simulink model "ATOM_simple_planning_simulator"  (R2026a)
settings: Solver=ode4  StopTime=50  FixedStep=0.01
StopFcn:
  | if exist('costmap_active','var') && ...
  |    exist('vehicle','var') && ...
  |    exist('parking_path','var') && ...
  |    ~isempty(parking_path)
  | 
  |     plotPlan(costmap_active, vehicle, parking_path);
  | else
  |     warning('No valid parking path is available for plotting.');
  | end
model workspace (MAT data in the model file):
  vehicle : object (value not decoded)
symbols that are objects in the model workspace (value not decoded): vehicle
undefined symbols (not defined in the file or in its folder): delta_f_LUT, gain4WS_LUT, k_ref_LUT, kappa_gain_BP, Ki, Kp, lateral, longitudinal, planning_validator, rr_gain_BP, rr_LUT, stanley, velocity_smoother
libraries: slpidlib x1, simulink x1
(part 7 of 7)

== matlab function ATOM_simple_planning_simulator/Plot vehicle1/SetStanleyTrajectory/Resample Trajectory ==
  data: trajectory_in input Bus: TrajectoryDataBus; trajectory_out output Bus: TrajectoryDataBus; resample_interval_dist input; nearest_seg_idx input; ego_offset_to_segment input
function trajectory_out = resampleTrajectoryByDistance( ...
    trajectory_in, ...
    resample_interval_dist, ...
    nearest_seg_idx, ...
    ego_offset_to_segment)


%% ============================================================
% RESAMPLE TRAJECTORY BY ARC LENGTH
%
% Equivalent to:
%
% MPCUtils::resampleMPCTrajectoryByDistance()
%
% Adapted for Stanley controller.
%
% Unlike MPC:
% - no MPCTrajectory conversion
% - no curvature resampling
% - no optimization variables
%
% The trajectory is directly interpolated in arc length.
%
% ATTENTION:
% 
% Resampling is not actuated in Simulink since in/out buses present fixed sizes.
% See NOTE at the end of this function.
%
% =============================================================


% N = length(trajectory_in.pose.position.x);
% 
% 
% if N < 2
% 
%     trajectory_out = trajectory_in;
%     return
% 
% end
% 
% 
% 
% %% ============================================================
% % Compute arc length
% % =============================================================
% 
% x = trajectory_in.pose.position.x;
% y = trajectory_in.pose.position.y;
% 
% 
% arc_length = zeros(N,1);
% 
% 
% for i = 2:N
% 
%     dx = x(i)-x(i-1);
%     dy = y(i)-y(i-1);
% 
%     arc_length(i)= ...
%         arc_length(i-1)+sqrt(dx^2+dy^2);
% 
% end
% 
% 
% 
% if isempty(arc_length)
% 
%     trajectory_out = trajectory_in;
%     return
% 
% end
% 
% 
% 
% %% ============================================================
% % Ego position along trajectory
% %
% % Equivalent to:
% %
% % input_arclength(nearest_seg_idx)
% % + ego_offset_to_segment
% %
% % =============================================================
% 
% 
% ego_s = arc_length(nearest_seg_idx) ...
%         + ego_offset_to_segment;
% 
% 
% ego_s = min(max(ego_s,0),arc_length(end));
% 
% 
% 
% %% ============================================================
% % Generate resampling points
% %
% % Same strategy as Autoware:
% % - backward from ego
% % - forward from ego
% %
% % =============================================================
% 
% 
% output_s = [];
% 
% 
% % backward direction
% 
% s = ego_s;
% 
% while s >= 0
% 
%     output_s = [s output_s]; %#ok<AGROW>
% 
%     s = s - resample_interval_dist;
% 
% end
% 
% 
% 
% % forward direction
% 
% s = ego_s + resample_interval_dist;
% 
% 
% while s < arc_length(end)
% 
%     output_s(end+1)=s; % #ok<AGROW>
% 
%     s = s + resample_interval_dist;
% 
% end
% 
% 
% 
% %% ============================================================
% % Interpolation
% % =============================================================
% 
% 
% x_new = interp1( ...
%     arc_length,...
%     x,...
%     output_s,...
%     'linear');
% 
% 
% 
% y_new = interp1( ...
%     arc_length,...
%     y,...
%     output_s,...
%     'linear');
% 
% 
% 
% z = trajectory_in.pose.position.z;
% 
% z_new = interp1( ...
%     arc_length,...
%     z,...
%     output_s,...
%     'linear');
% 
% 
% 
% %% ============================================================
% % Quaternion / yaw interpolation
% %
% % Stanley works with yaw.
% % Therefore interpolate yaw and rebuild quaternion.
% %
% % =============================================================
% 
% 
% yaw = QuaternionToYaw( ...
%     trajectory_in.pose.orientation.qx,...
%     trajectory_in.pose.orientation.qy,...
%     trajectory_in.pose.orientation.qz,...
%     trajectory_in.pose.orientation.qw);
% 
% 
% 
% % avoid discontinuity
% 
% yaw = unwrap(yaw);
% 
% 
% 
% yaw_new = interp1( ...
%     arc_length,...
%     yaw,...
%     output_s,...
%     'linear');
% 
% 
% 
% %% ============================================================
% % Velocity interpolation
% %
% % Autoware uses linear interpolation
% % =============================================================
% 
% 
% vel_new = interp1( ...
%     arc_length,...
%     trajectory_in.longitudinal_velocity_mps,...
%     output_s,...
%     'linear');
% 
% 
% 
% lat_vel_new = interp1( ...
%     arc_length,...
%     trajectory_in.lateral_velocity_mps,...
%     output_s,...
%     'linear');
% 
% 
% 
% acc_new = interp1( ...
%     arc_length,...
%     trajectory_in.acceleration_mps2,...
%     output_s,...
%     'linear');
% 
% 
% 
% %% ============================================================
% % Build output structure
% % =============================================================
% 
% 
% M = length(output_s);
% 
% 
% trajectory_out.pose.position.x = x_new;
% trajectory_out.pose.position.y = y_new;
% trajectory_out.pose.position.z = z_new;
% 
% 
% 
% [qx,qy,qz,qw] = yawToQuaternion(yaw_new);
% 
% 
% 
% trajectory_out.pose.orientation.qx = qx;
% trajectory_out.pose.orientation.qy = qy;
% trajectory_out.pose.orientation.qz = qz;
% trajectory_out.pose.orientation.qw = qw;
% 
% 
% 
% trajectory_out.longitudinal_velocity_mps = vel_new;
% 
% trajectory_out.lateral_velocity_mps = lat_vel_new;
% 
% trajectory_out.acceleration_mps2 = acc_new;
% 
% 
% 
% % steering values are kept
% 
% trajectory_out.front_wheel_angle_rad = ...
%     interp1( ...
%     arc_length,...
%     trajectory_in.front_wheel_angle_rad,...
%     output_s,...
%     'linear');
% 
% 
% trajectory_out.rear_wheel_angle_rad = ...
%     interp1( ...
%     arc_length,...
%     trajectory_in.rear_wheel_angle_rad,...
%     output_s,...
%     'linear');
% 
% 


%% ============================================================
% NOTE (Simulink Implementation)
%
% The trajectory resampling algorithm reported above is equivalent
% to the implementation adopted by Autoware.
%
% However, the main objective of the present work is the development
% and validation of the 4WS Stanley Controller rather than the
% trajectory preprocessing module.
%
% Since Simulink requires fixed-size bus signals, the resampled
% trajectory is not generated in the simulation model.
%
% The original input trajectory is therefore directly propagated to
% the controller, preserving its fixed dimension and avoiding the
% introduction of variable-length signals.
%
% Consequently, the following assignment overwrites the resampled
% trajectory computed above.
%
% ============================================================

trajectory_out = trajectory_in;

end

== matlab function ATOM_simple_planning_simulator/Plot vehicle1/SetStanleyTrajectory/calcLongOffsetToSegment ==
  data: seg_idx input; ego_pose input; trajectory input Bus: TrajectoryDataBus; ego_offset_to_segment output
function ego_offset_to_segment = calcLongOffsetToSegment(seg_idx, ego_pose, trajectory)

ego_offset_to_segment = calcLongitudinalOffsetToSegment(trajectory, seg_idx, ego_pose);

end

== matlab function ATOM_simple_planning_simulator/Plot vehicle1/SetStanleyTrajectory/findFirstNearestSegmentIndexWithSoftConstraints ==
  data: trajectory input; dist_threshold input; yaw_threshold input; nearest_seg_idx output; pose input
function nearest_seg_idx = findNearestSegmentIndexWithSoftConstraints( ...
    trajectory, dist_threshold, yaw_threshold, pose)


%% Step 1:
% Find nearest point index

nearest_idx = findFirstNearestIndexWithSoftConstraints( ...
    trajectory, ...
    pose, ...
    dist_threshold, ...
    yaw_threshold);


N = length(trajectory.pose.position.x);


%% Step 2:
% Convert point index into segment index

% First point
if nearest_idx == 1

    nearest_seg_idx = 1;
    return

end


% Last point
if nearest_idx == N

    nearest_seg_idx = N-1;
    return

end



%% Step 3:
% Determine whether ego lies before or after nearest point
%
% Equivalent to Autoware:
%
% signed_length =
% calcLongitudinalOffsetToSegment(points,
%                                 nearest_idx,
%                                 pose.position)


signed_length = calcLongitudinalOffsetToSegment( ...
    trajectory,...
    nearest_idx,...
    pose);



%% Step 4:
% Choose segment

if signed_length <= 0

    % ego is before nearest point
    %
    % Autoware:
    % return nearest_idx - 1;

    nearest_seg_idx = nearest_idx - 1;


else

    % ego is after nearest point
    %
    % Autoware:
    % return nearest_idx;

    nearest_seg_idx = nearest_idx;

end


end

== matlab function ATOM_simple_planning_simulator/Parking Scenario/MATLAB Function ==
  data: segment_done input; segment_request output; segment_count input; maneuver_complete output
function [segment_request, maneuver_complete] = ...
    segmentManager(segment_done, segment_count)
%SEGMENTMANAGER
% Advance exactly once when the current segment is completed.

persistent active_segment previous_done complete_latched

if isempty(active_segment)
    active_segment  = 1.0;
    previous_done   = false;
    complete_latched = false;
end

% Convert the inputs into known scalar types.
done_now = logical(segment_done);
count = max(0.0, floor(double(segment_count)));

% Protect against an active index larger than the available count.
if count > 0 && active_segment > count
    active_segment = count;
end

% Detect only the transition from not-done to done.
done_rising_edge = done_now && ~previous_done;

if done_rising_edge && count > 0

    if active_segment < count

        % Another segment exists.
        active_segment = active_segment + 1.0;

    else

        % The final segment has been completed.
        complete_latched = true;

    end
end

previous_done = done_now;

segment_request  = active_segment;
maneuver_complete = complete_latched;
end

== matlab function ATOM_simple_planning_simulator/parking_velocity_smoother/MATLAB Function ==
  data: trajectory_in input Bus: TrajectoryDataBus size=1; trajectory_out output Bus: TrajectoryDataBus size=1
function trajectory_out = parkingVelocitySmoother(trajectory_in)
%#codegen
%
% Generate the longitudinal velocity and acceleration reference
% for one forward or reverse parking segment.

% Preserve all fields of the original trajectory bus.
trajectory_out = trajectory_in;

% The parking trajectory contains exactly 100 points.
N = 100;

%% 1. Velocity-profile parameters

v_max       = 2.00;   % desired maximum parking speed [m/s]
a_accel_max = 1.00;   % from velocity_smoother.max_acc
% Plan the trajectory using gentler braking than the controller can
% physically command. The remaining 0.50 m/s^2 provides correction margin
% for tracking error, actuator delay, and acceleration lag.
a_decel_max = 0.50;   % planned braking magnitude [m/s^2]

% Existing lateral-acceleration limit from velocity_smoother_params.m.
a_lat_max = 1.00;     % maximum lateral acceleration [m/s^2]

% Existing curvature-calculation distance from
% velocity_smoother_params.m.
curvature_calculation_distance = 2.00;   % [m]

%% 2. Read the trajectory data

px = trajectory_in.pose.position.x;
py = trajectory_in.pose.position.y;

rear_angle = trajectory_in.rear_wheel_angle_rad;

% At this stage, the incoming velocity is used only to determine
% whether the segment is forward or reverse.
raw_velocity = trajectory_in.longitudinal_velocity_mps;

%% 3. Determine the segment direction

% Default to forward if no nonzero direction can be found.
gear = 1.0;

for k = 1:N
    if abs(raw_velocity(k)) > 1e-6
        gear = sign(raw_velocity(k));
        break;
    end
end

%% 4. Calculate distance between consecutive trajectory points

ds = zeros(N-1,1);
path_length = 0.0;

for k = 1:N-1
    dx = px(k+1) - px(k);
    dy = py(k+1) - py(k);

    ds(k) = hypot(dx,dy);
    path_length = path_length + ds(k);
end

%% 5. Calculate trajectory curvature

% pathToTrajectory resamples the segment at approximately equal
% distances, so an index separation can represent the requested
% curvature-calculation distance.

point_interval = path_length / (N-1);

idx_dist = 1;

if point_interval > 1e-6
    idx_dist = floor( ...
        curvature_calculation_distance / point_interval);
end

% Three curvature points must remain inside the trajectory.
max_idx_dist = floor((N-1)/2);

idx_dist = max(1,min(idx_dist,max_idx_dist));

curvature = zeros(N,1);

for k = 2:N-1

    idx_prev = k - min(idx_dist,k-1);
    idx_next = k + min(idx_dist,N-k);

    x1 = px(idx_prev);
    y1 = py(idx_prev);

    x2 = px(k);
    y2 = py(k);

    x3 = px(idx_next);
    y3 = py(idx_next);

    d12 = hypot(x2-x1,y2-y1);
    d23 = hypot(x3-x2,y3-y2);
    d31 = hypot(x1-x3,y1-y3);

    denominator = d12*d23*d31;

    if abs(denominator) > 1e-10

        curvature(k) = 2.0 * ( ...
            (x2-x1)*(y3-y1) - ...
            (y2-y1)*(x3-x1)) / denominator;

    else

        % Degenerate or repeated trajectory points.
        curvature(k) = 0.0;

    end
end

% Complete the two boundary values.
curvature(1) = curvature(2);
curvature(N) = curvature(N-1);

%% 6. Build the speed ceiling

% Begin with the requested maximum parking speed.
speed_limit = v_max * ones(N,1);

% Reduce the speed wherever the trajectory curvature would cause the
% lateral acceleration to exceed a_lat_max.
%
% Current 4WS model relation:
%
%     a_lat = vx^2 * curvature / cos(delta_r)
%
% Therefore:
%
%     vx_max = sqrt(a_lat_max*cos(delta_r)/abs(curvature))

for k = 1:N

    kappa = abs(curvature(k));

    if kappa > 1e-6

        cos_rear = cos(rear_angle(k));

        % Numerical protection. With the present steering limits,
        % cos(rear_angle) should remain positive.
        if cos_rear < 1e-6
            cos_rear = 1e-6;
        end

        v_lateral_max = sqrt( ...
            a_lat_max*cos_rear/kappa);

        % The final local ceiling is the smaller of:
        %   1. the 2 m/s parking limit;
        %   2. the curvature-based lateral limit.
        speed_limit(k) = min( ...
            speed_limit(k), ...
            v_lateral_max);
    end
end

%% 7. Backward pass: ensure that the vehicle can stop

speed_backward = speed_limit;

% Every parking segment ends at rest.
speed_backward(N) = 0.0;

for k = N-1:-1:1

    % Maximum speed at point k from which the vehicle can still
    % brake to speed_backward(k+1).
    reachable_speed = sqrt( ...
        speed_backward(k+1)^2 + ...
        2.0*a_decel_max*ds(k));

    speed_backward(k) = min( ...
        speed_backward(k), ...
        reachable_speed);
end

%% 8. Forward pass: enforce the acceleration limit

speed_magnitude = speed_backward;

% Every segment starts at rest, including after a gear reversal.
speed_magnitude(1) = 0.0;

for k = 2:N

    % Maximum speed reachable from the previous point without
    % exceeding a_accel_max.
    reachable_speed = sqrt( ...
        speed_magnitude(k-1)^2 + ...
        2.0*a_accel_max*ds(k-1));

    speed_magnitude(k) = min( ...
        speed_backward(k), ...
        reachable_speed);
end

%% 9. Calculate the compatible acceleration reference

acceleration_magnitude = zeros(N,1);

for k = 1:N-1

    if ds(k) > 1e-6

        acceleration_magnitude(k) = ...
            (speed_magnitude(k+1)^2 - ...
             speed_magnitude(k)^2) / ...
            (2.0*ds(k));

    else

        % Protect against duplicate consecutive points.
        acceleration_magnitude(k) = 0.0;

    end
end

% The vehicle remains stopped at the segment endpoint.
acceleration_magnitude(N) = 0.0;

%% 10. Apply the forward or reverse sign

trajectory_out.longitudinal_velocity_mps = ...
    gear*speed_magnitude;

trajectory_out.acceleration_mps2 = ...
    gear*acceleration_magnitude;

end

== matlab function ATOM_simple_planning_simulator/Subsystem/parkingLongitudinalController ==
  data: tx input; a_cmd output; ty input; tvx input; tax input; s_now input; vx input; longitudinal_mode input; a_ref_out output
function [a_cmd,a_ref_out] = parkingLongitudinalController( ...
    tx, ty, tvx, tax, s_now, vx, longitudinal_mode)
%#codegen
%
% Independent longitudinal parking controller.
%
% Inputs:
%   tx, ty  : trajectory position arrays
%   tvx     : signed velocity reference array
%   tax     : signed acceleration feedforward array
%   s_now   : current progress along the trajectory
%   vx      : measured longitudinal velocity
%   longitudinal_mode:
%             0 = normal profile tracking
%             1 = terminal creep
%             2 = stop
%
% Output:
%   a_cmd   : commanded longitudinal acceleration

N = 100;

% Normal velocity-tracking gain.
Kp = 1.0;

% Stronger gain used only when stopping at a segment endpoint.
% With the 1 m/s^2 command limit, this requests maximum braking whenever
% the speed magnitude is greater than or equal to 0.20 m/s.
Kp_stop = 5.0;

% Existing velocity-smoother longitudinal acceleration limit.
a_cmd_limit = 1.0;

terminal_creep_speed = 0.05;

%% Construct trajectory arc length

s = zeros(N,1);

for k = 2:N
    s(k) = s(k-1) + hypot( ...
        tx(k)-tx(k-1), ...
        ty(k)-ty(k-1));
end

%% Read the feedforward references at the current progress

v_ref = lookupS(s,tvx,s_now);
a_ref = lookupS(s,tax,s_now);

%% Determine the forward or reverse direction

gear = 1.0;

for k = 1:N
    if abs(tvx(k)) > 1e-6
        gear = sign(tvx(k));
        break;
    end
end

%% Apply the maneuver-supervisor mode
%% Apply the maneuver-supervisor mode

% Use the normal tracking gain unless stop mode selects the stronger gain.
Kp_active = Kp;

if longitudinal_mode == 2.0

    % Stop mode.
    % Drive the measured velocity firmly toward zero.
    v_ref = 0.0;
    a_ref = 0.0;
    Kp_active = Kp_stop;

elseif longitudinal_mode == 1.0

    % Very slow endpoint correction.
    v_ref = gear*terminal_creep_speed;
    a_ref = 0.0;

end

% Acceleration reference currently selected at the vehicle's progress.
a_ref_out = a_ref;
%% Feedforward plus velocity-error correction

%% Feedforward plus velocity-error correction

speed_error = v_ref - vx;

% Express the measured and reference velocities in the direction of the
% current segment. Positive means movement in the intended gear direction.
speed_in_gear = gear * vx;
reference_speed_in_gear = gear * v_ref;
feedforward_in_gear = gear * a_ref;

% A negative feedforward value means braking.
%
% Apply braking feedforward only while the vehicle is moving faster than
% its reference. Once the vehicle is at or below the reference speed,
% remove the braking feedforward and let the velocity feedback correct it.
%
% This also prevents the controller from intentionally accelerating the
% vehicle in the opposite direction before the segment manager authorizes
% a gear change.
a_feedforward = a_ref;

if feedforward_in_gear < 0.0 && ...
        speed_in_gear <= reference_speed_in_gear

    a_feedforward = 0.0;

end

a_unsaturated = ...
    a_feedforward + Kp_active*speed_error;

a_cmd = max( ...
    -a_cmd_limit, ...
    min(a_cmd_limit,a_unsaturated));

end

%--------------------------------------------------------------------------
function value = lookupS(sv,vv,s_query)
% Linear interpolation of a trajectory quantity by path distance.

n = numel(sv);
value = vv(n);

if s_query <= sv(1)
    value = vv(1);
    return;
end

if s_query >= sv(n)
    return;
end

for k = 1:n-1

    if s_query <= sv(k+1)

        ds = sv(k+1)-sv(k);

        if ds < 1e-12
            value = vv(k+1);
        else
            ratio = (s_query-sv(k))/ds;
            value = vv(k) + ratio*(vv(k+1)-vv(k));
        end

        return;
    end
end

end

== matlab function ATOM_simple_planning_simulator/velocity_smoother_node/ApplySteeringRateLimit - velocity_smoother_node/ApplyPreProcess ==
  data: input input Bus: TrajectoryDataBus; use_resempling input boolean; output output Bus: TrajectoryDataBus; points_interval input double
function output = applyPreProcess(input, use_resempling, points_interval)

% ApplyPreProcess
%
% This function reproduces the first stage of Autoware
% SmootherBase::applyPreProcess().
%
% In Autoware, when resampling is enabled, the input trajectory
% is interpolated with a constant spatial interval.
%
% In this Simulink implementation the resampling stage is omitted
% (use_resempling == false)
% The original trajectory points are directly forwarded to the next block.
%

output = input;

end

== matlab function ATOM_simple_planning_simulator/Parking Scenario/Costmap generation: obstacle1/MATLAB Function ==
  settings: updateMethod=DISCRETE
  data: costmap output Bus: OccupancyGridBus; start_pose output; goal_pose output; veh input
function [costmap, start_pose, goal_pose] = costmapOffsetDock(veh)
%COSTMAPOFFSETDOCK  A short, angled parking bay beside a narrow aisle.
% Paste into a duplicate of an existing costmap MATLAB Function block.
% Inputs/outputs and the 234-by-234 int8 payload match the current model.
% Poses refer to the rear-axle centre; headings are in radians.

%% Map and scene dimensions [m]
res = 0.20;
W = 234;
H = 234;
origin_x = -(W/2)*res;
origin_y = -(H/2)*res;

aisle_width = 3.20;
aisle_x_min = -8.9;
aisle_x_max =  7.1;
aisle_center_y = 0.10;

bay_length = 4.30;
bay_width  = 3.40;
bay_angle  = 15*pi/180;
bay_center_x = 0.0;
bay_center_y = 2.70;

%% Rear-axle start and goal poses
start_pose = [-5.0, 0.0, pi];

% The bay centre is a BODY-centre position, not a rear-axle position.
body_center_from_rear_axle = (veh(3) + veh(5) - veh(6))/2;
goal_pose = [ ...
    bay_center_x - body_center_from_rear_axle*cos(bay_angle), ...
    bay_center_y - body_center_from_rear_axle*sin(bay_angle), ...
    bay_angle];

%% Occupancy grid
% Stateless: each call reflects the dimensions above, without a cached map.
[IX,IY] = meshgrid(0:W-1,0:H-1);
X = origin_x + IX*res;
Y = origin_y + IY*res;

% Avoid asymmetric inclusion of boundary points due to floating-point error.
tol = 1e-9;
% These walls coincide with cell edges. Include only complete free cells.
% The start is 0.10 m below the aisle centreline.
aisle = X >= aisle_x_min+res/2-tol & X <= aisle_x_max-res/2+tol & ...
        abs(Y-aisle_center_y) <= aisle_width/2-res/2+tol;

% Coordinates along/across the angled bay.
dx = X-bay_center_x;
dy = Y-bay_center_y;
along  =  cos(bay_angle)*dx + sin(bay_angle)*dy;
across = -sin(bay_angle)*dx + cos(bay_angle)*dy;
bay = abs(along) <= bay_length/2+tol & ...
      abs(across) <= bay_width/2+tol;

% Free space is the union of the aisle and bay. Everything else is occupied.
% No obstacle inflation is added here. The planner handles its ego margin.
occupied = ~(aisle | bay);

%% Existing OccupancyGrid bus format
costmap.info.resolution = res;
costmap.info.width  = uint32(W);
costmap.info.height = uint32(H);
costmap.info.origin.position.x = origin_x;
costmap.info.origin.position.y = origin_y;
costmap.info.origin.position.z = 0;
costmap.info.origin.orientation.x = 0;
costmap.info.origin.orientation.y = 0;
costmap.info.origin.orientation.z = 0;
costmap.info.origin.orientation.w = 1;
costmap.data = int8(occupied).*int8(100);
end

== matlab function ATOM_simple_planning_simulator/Parking Scenario/Costmap generation: obstacle2/MATLAB Function ==
  settings: updateMethod=DISCRETE
  data: costmap output Bus: OccupancyGridBus; start_pose output; goal_pose output; veh input
function [costmap, start_pose, goal_pose] = costmapUndergroundParking(veh)
%COSTMAPUNDERGROUNDPARKING  Realistic reverse parking in a double-row garage.
% The target is the empty bay at x = 0 in the upper row. Parked vehicles
% surround it, an opposing row limits the aisle, and a structural column is
% located beside the entrance. Poses refer to the rear-axle centre.

%% Fixed OccupancyGrid dimensions used by the current model
res = 0.20;
W = 234;
H = 234;
origin_x = -(W/2)*res;
origin_y = -(H/2)*res;
[IX,IY] = meshgrid(0:W-1,0:H-1);
X = origin_x + IX*res;
Y = origin_y + IY*res;

%% Garage geometry [m]
aisle_width = 6.50;       % clear nominal two-way manoeuvring aisle
parking_depth = 5.20;
bay_pitch = 3.20;         % centre-to-centre bay spacing
parked_length = 4.60;     % physical parked vehicle, no inflation here
parked_width = 2.00;
pillar_size = 0.40;

garage_x_min = -11.0;
garage_x_max =  11.0;
garage_y_min = -(aisle_width/2 + parking_depth);
garage_y_max =  (aisle_width/2 + parking_depth);

% Start occupied and carve out the garage floor.
occupied = true(H,W);
garage_floor = X >= garage_x_min & X <= garage_x_max & ...
               Y >= garage_y_min & Y <= garage_y_max;
occupied(garage_floor) = false;

%% Parked vehicles
row_y = aisle_width/2 + parking_depth/2;
bay_x = (-3:3)*bay_pitch;

for k = 1:numel(bay_x)
    % Upper row: leave the centre bay empty.
    if k ~= 4
        top_car = abs(X-bay_x(k)) <= parked_width/2 & ...
                  abs(Y-row_y) <= parked_length/2;
        occupied(top_car) = true;
    end

    % Opposing row: all bays occupied.
    bottom_car = abs(X-bay_x(k)) <= parked_width/2 & ...
                 abs(Y+row_y) <= parked_length/2;
    occupied(bottom_car) = true;
end

%% Structural column beside the target bay entrance
pillar_x = bay_pitch/2;
pillar_y = aisle_width/2 + pillar_size/2 + 0.10;
pillar = abs(X-pillar_x) <= pillar_size/2 & ...
         abs(Y-pillar_y) <= pillar_size/2;
occupied(pillar) = true;

%% Parking task
% The vehicle begins beside the target bay, as it would after approaching
% through the aisle, and reverses into the upper-row space.
start_pose = [-5.0, 0.0, pi/2];
goal_pose = [0.0, row_y, -pi/2];

%% Existing OccupancyGrid bus format
costmap.info.resolution = res;
costmap.info.width = uint32(W);
costmap.info.height = uint32(H);
costmap.info.origin.position.x = origin_x;
costmap.info.origin.position.y = origin_y;
costmap.info.origin.position.z = 0;
costmap.info.origin.orientation.x = 0;
costmap.info.origin.orientation.y = 0;
costmap.info.origin.orientation.z = 0;
costmap.info.origin.orientation.w = 1;
costmap.data = int8(occupied).*int8(100);

% veh is intentionally kept as the input because the surrounding subsystem
% already supplies the 29-element vehicle vector and all costmap blocks use
% the same interface. Geometry above represents other parked vehicles.
if numel(veh) < 8
    error('costmapUndergroundParking:VehSize', ...
        'veh must be the complete vehicle-parameter vector.');
end
end
